simulink subsystem "rss_pmsm_motor_simscape_deltaconn"  (R2024a)
settings: Solver=VariableStepAuto  StartTime=0.0  StopTime=10.0  RelTol=1e-3
undefined symbols (not defined in the file): parMotMdlPolePairNum
libraries: nesl_utility x11, fl_lib x10, ee_lib x2, mcbcontrolslib x1
settings Model: Creator=CAV2OFO  LastModifiedBy=pav2ofo
settings OptimizationCC: ReuseModelBlockBuffer=off
settings RTWCC: GPUComputeCapability=3.5

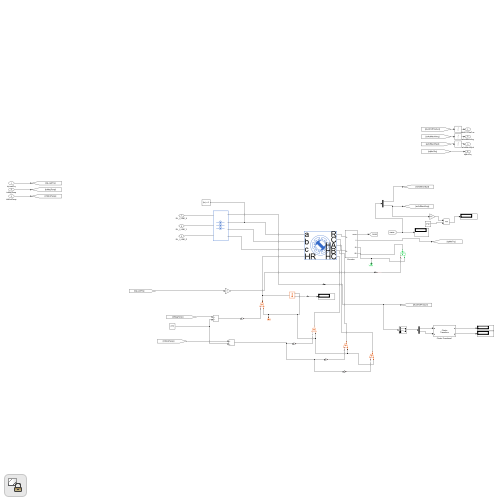
[thumbnail: Simulink's stored preview of the top-level diagram]
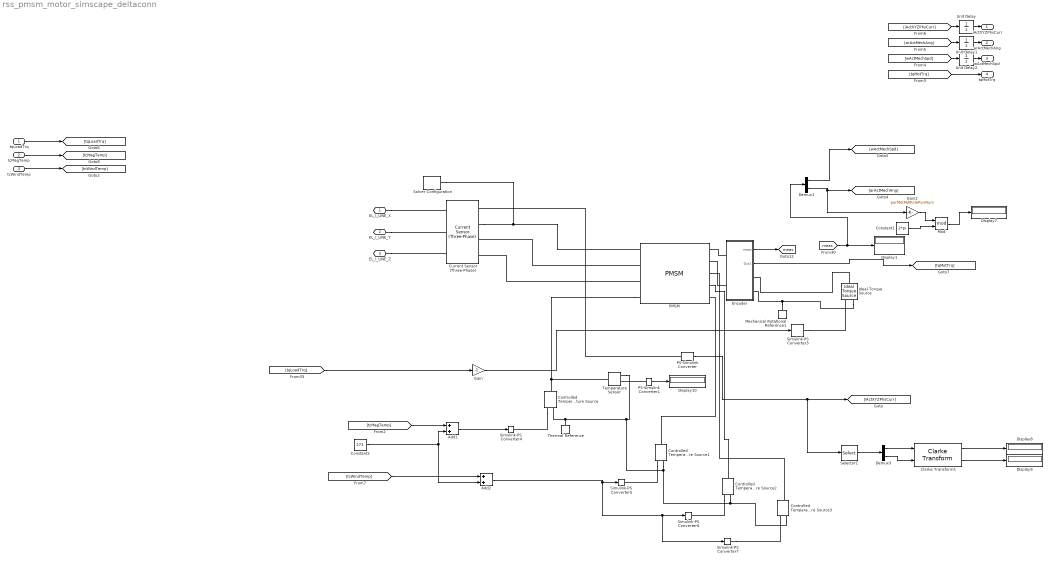
== system rss_pmsm_motor_simscape_deltaconn ==
  tqLoadTrq : Inport
  tcMagTemp : Inport  Port=2
  tcWindTemp : Inport  Port=3
  Add1 : Sum
  Add2 : Sum
  Clarke Transform1 : mcbcontrolslib/Clarke Transform  VariantControl=Variant2  PhaseInput=Two inputs  EnPowerInv=off
      settings: LibrarySourceBlock=mcbhdllib/Controls/Math Transforms/Clarke Transform
  Constant1 : Constant  Value=2*pi
  Constant2 : Constant  Value=273
  Controlled Temperature Source{,1..3} (4 alike) : fl_lib/Thermal/Thermal Sources/Controlled Temperature Source
  Current Sensor (Three-Phase) : ee_lib/Sensors & Transducers/Current Sensor (Three-Phase)
      settings: InternalSimscapePortConfiguration="{\"Bottom\":[],\"Left\":[{\"id\":\"a1\",\"label\":\"a1\",\"type\":\"foundation.electrical.electrical\"},{\"id\":\"b1\",\"label\":\"b1\",\"type\":\"foundation.electrical.electrical\"},{\"id\":\"c1\",\"label\":\"c1\",\"type\":\"foundation.electrical.electrical\"}],\"Right\":[{\"id\":\"I_output\",\"label\":\"I\",\"type\":\"output\"},{\"id\":\"a2\",\"label\":\"a2\",\"type\":\"foundation.electrical.electrical\"},{\"id\":\"b2\",\"label\":\"b2\",\"type\":\"foundation.electrical.electrical\"},{\"id\":\"c2\",\"label\":\"c2\",\"type\":\"foundation.electrical.electrical\"}],\"Top\":[]}"
  Demux1 : Demux  Outputs=2
  Demux3 : Demux  Outputs=2
  Display{1,7..10} (5 alike) : Display
  Encoder : Subsystem
  Gain : Gain  Gain=-1
  Gain2 : Gain  Gain=parMotMdlPolePairNum
  Ideal Torque Source : fl_lib/Mechanical/Mechanical Sources/Ideal Torque Source
  Mechanical Rotational Reference1 : fl_lib/Mechanical/Rotational Elements/Mechanical Rotational Reference
  Mod : Math  Operator=mod
  PMSM : ee_lib/Electromechanical/Permanent Magnet/PMSM  port_option=ee.enum.threePhasePort.expanded  winding_type=ee.enum.statorconnection.delta  machine_param=ee.enum.pmsm.parameterization.constant  nPolePairs=parMotMdlPolePairNum  pmflux_param=ee.enum.pmflux.fluxlinkage  pm_flux_linkage=parMotMdlPermMagFlux Wb  torque_constant=0.18 N*m/A  back_emf_constant=0.18 V*s/rad  stator_param=ee.enum.statorparam.LdLqL0  Ld=parMotMdlDirIndc H  Lq=parMotMdlQdrtIndc H  idVec=[-200, 0, 200] A  iqVec=[-200, 0, 200] A  LdMatrix=0.0002 * ones(3, 3) H  LqMatrix=0.0002 * ones(3, 3) H  PmMatrix=0.1 * ones(3, 3) Wb  ktMatrix=0.18 * ones(3, 3) N*m/A  keMatrix=0.18 * ones(3, 3) V*s/rad  L0=0 H  Ls=0.0002 H  Lm=-0.00002 H  Ms=0.00002 H  Rs=parMotMdlPhsRstn Ohm  zero_sequence=ee.enum.park.zerosequence.exclude  axes_param=ee.enum.rotorangle.daxis  loss_param=ee.enum.ironloss.none  losses_oc=[0, 0, 0] W  losses_sc=[0, 0, 0] W  f_losses=60 Hz  Isc_losses=95 A  J=1.652E-5 kg*m^2  lam=double(7.9577471545947675E-5)*pi/30 N*m*s/rad  i_d_specify=on  i_d_priority=None  i_d=0.1 A  i_d_nominal_specify=off  i_d_nominal_value=1  i_d_nominal_unit=A  i_q_specify=on  i_q_priority=None  i_q=0.1 A  i_q_nominal_specify=off  i_q_nominal_value=1  i_q_nominal_unit=A  torque_specify=off  torque_priority=None  torque=0 N*m  torque_nominal_specify=off  torque_nominal_value=1  torque_nominal_unit=N*m  angular_velocity_specify=off  angular_velocity_priority=High  angular_velocity=0 rpm  angular_velocity_nominal_specify=off  angular_velocity_nominal_value=1  angular_velocity_nominal_unit=rpm  angular_position_specify=off  angular_position_priority=High  angular_position=0 deg  angular_position_nominal_specify=off  angular_position_nominal_value=1  angular_position_nominal_unit=deg  alpha=parMotRstnTempCoef 1/K  alpha_flux=parMotMdlMagTempCoef 1/K  Tmeas=25 degC  stator_thermal_mass=100 J/K  rotor_thermal_mass=200 J/K  Rm_percent_rotor=90  Rd_percent_rotor=30  temperatureA_specify=on  temperatureA_priority=Low  temperatureA=25 degC  temperatureA_nominal_specify=off  temperatureA_nominal_value=1  temperatureA_nominal_unit=degC  temperatureB_specify=on  temperatureB_priority=Low  temperatureB=25 degC  temperatureB_nominal_specify=off  temperatureB_nominal_value=1  temperatureB_nominal_unit=degC  temperatureC_specify=on  temperatureC_priority=Low  temperatureC=25 degC  temperatureC_nominal_specify=off  temperatureC_nominal_value=1  temperatureC_nominal_unit=degC  temperatureR_specify=on  temperatureR_priority=Low  temperatureR=25 degC  temperatureR_nominal_specify=off  temperatureR_nominal_value=1  temperatureR_nominal_unit=degC
      settings: InternalSimscapePortConfiguration="{\"Bottom\":[],\"Left\":[{\"id\":\"a\",\"label\":\"a\",\"type\":\"foundation.electrical.electrical\"},{\"id\":\"b\",\"label\":\"b\",\"type\":\"foundation.electrical.electrical\"},{\"id\":\"c\",\"label\":\"c\",\"type\":\"foundation.electrical.electrical\"},{\"id\":\"HR\",\"label\":\"HR\",\"type\":\"foundation.thermal.thermal\"}],\"Right\":[{\"id\":\"R\",\"label\":\"R\",\"type\":\"foundation.mechanical.rotational.rotational\"},{\"id\":\"C\",\"label\":\"C\",\"type\":\"foundation.mechanical.rotational.rotational\"},{\"id\":\"HA\",\"label\":\"HA\",\"type\":\"foundation.thermal.thermal\"},{\"id\":\"HB\",\"label\":\"HB\",\"type\":\"foundation.thermal.thermal\"},{\"id\":\"HC\",\"label\":\"HC\",\"type\":\"foundation.thermal.thermal\"}],\"Top\":[]}"
  PS-Simulink Converter : nesl_utility/PS-Simulink Converter  PhysicalDomain=network_engine_domain  SubClassName=ps_output  LeftPortType=input  RightPortType=output  PseudoPeriodic=off  Frequencies=[]  VectorFormat=1-D array  Unit=A  AffineConversion=off
  PS-Simulink Converter1 : nesl_utility/PS-Simulink Converter  PhysicalDomain=network_engine_domain  SubClassName=ps_output  LeftPortType=input  RightPortType=output  PseudoPeriodic=off  Frequencies=[]  VectorFormat=inherit  Unit=inherit  AffineConversion=off
  Selector1 : Selector  InputPortWidth=3  IndexOptions=Index vector (dialog)  Indices=[1 2]  OutputSizes=1
  Simulink-PS Converter3 : nesl_utility/Simulink-PS Converter  PhysicalDomain=network_engine_domain  SubClassName=ps_input  LeftPortType=input  RightPortType=output  PseudoPeriodic=off  Frequencies=[]  NoiseDistribution=none  NoiseParameters=[]  Unit=1  AffineConversion=off  FilteringAndDerivatives=zero  SimscapeFilterOrder=1  InputFilterTimeConstant=.001  UdotUserProvided=0
  Simulink-PS Converter{4..7} (4 alike) : nesl_utility/Simulink-PS Converter  PhysicalDomain=network_engine_domain  SubClassName=ps_input  LeftPortType=input  RightPortType=output  PseudoPeriodic=off  Frequencies=[]  NoiseDistribution=none  NoiseParameters=[]  Unit=1  AffineConversion=off  FilteringAndDerivatives=filter  SimscapeFilterOrder=1  InputFilterTimeConstant=0.001  UdotUserProvided=0
  Solver Configuration : nesl_utility/Solver Configuration  PhysicalDomain=network_engine_domain  SubClassName=solver  LeftPortType=input  RightPortType=generic  Tones=[]  Harmonics=[]  SimulateNoise=off  Profile=off  UseLocalSampling=off  EnableSwitchedLinearOptims=on  FrequencyDomain=off  UseCCode=off  RelTol=0.001  AbsTol=0.001  MinStep=1e-09  ToWorkspace=off  RevertToSquareIcSolve=off  NumHomotopyIterations=100  PhasorMode=off  PhasorModeNumHarmonics=1  ConsistencySolver=NEWTON_XTOL_AFTER_FTOL  IndexReductionMethod=DerivativeReplacement  DoDC=off  ResidualTolerance=1e-09  ConsistencyTolSource=GLOBAL  ConsistencyAbsTol=0.001  ConsistencyRelTol=0.001  ConsistencyTolFactor=0.001  UseLocalSolver=on  LocalSolverChoice=NE_BACKWARD_EULER_ADVANCER  ResolveIndetEquations=on  FunctionEvalNumThread=1  LocalSolverSampleTime=cstMotorMdlSampTime  DoFixedCost=on  MaxNonlinIter=3  MaxModeIter=2  ComputeImpulses=off  ImpulseIterations=2  LinearAlgebra=auto  LinearAlgebraNumThread=0  EquationFormulation=NE_TIME_EF  DelaysMemoryBudget=1024  AutomaticFiltering=on  FilteringTimeConstant=0.001  PartitionStorageMethod=AS_NEEDED  PartitionMemoryBudget=1024  PartitionMethod=ROBUST  MultibodyUseLocalSolver=off  MultibodyLocalSolverChoice=ODE1  MultibodyLocalSolverSampleTime=0.001
  Temperature Sensor : fl_lib/Thermal/Thermal Sensors/Temperature Sensor  temperature_measure=foundation.enum.MeasurementReference.difference
  Thermal Reference : fl_lib/Thermal/Thermal Elements/Thermal Reference
  Unit Delay : UnitDelay  SampleTime=-1  HasFrameUpgradeWarning=on
  Unit Delay1 : UnitDelay  SampleTime=-1  HasFrameUpgradeWarning=on
  Unit Delay2 : UnitDelay  SampleTime=-1  HasFrameUpgradeWarning=on
  EL_I_LINE_X : PMIOPort  Side=Left
  EL_I_LINE_Y : PMIOPort  Port=2  Side=Left
  EL_I_LINE_Z : PMIOPort  Port=3  Side=Left
  iActXYZPhsCurr : Outport
  arActMechAng : Outport  Port=2
  wActMechSpd : Outport  Port=3
  tqMotTrq : Outport  Port=4
  tag scope: meas=global
  wires:
  Encoder/1(meas) -> [meas]
  Add2/1 -> Simulink-PS Converter7/1, Simulink-PS Converter6/1, Simulink-PS Converter5/1
  Clarke Transform1/1 -> Display8/1
  [tqMotTrq] -> tqMotTrq/1
  tqLoadTrq/1 -> [tqLoadTrq]
  Mod/1 -> Display7/1
  Constant2/1 -> Add2/2, Add1/2
  tcMagTemp/1 -> [tcMagTemp]
  [tcWindTemp] -> Add2/1
  Clarke Transform1/2 -> Display9/1
  Unit Delay1/1 -> arActMechAng/1
  Add1/1 -> Simulink-PS Converter4/1
  Gain/1 -> Simulink-PS Converter3/1
  Demux1/1 -> [wActMechSpd]
  PS-Simulink Converter1/1 -> Display10/1
  Unit Delay2/1 -> wActMechSpd/1
  Encoder/2(Out1) -> [tqMotTrq]
  tcWindTemp/1 -> [tcWindTemp]
  Demux1/2 -> Gain2/1, [arActMechAng]
  Unit Delay/1 -> iActXYZPhsCurr/1
  Constant1/1 -> Mod/2
  Gain2/1 -> Mod/1
  [tcMagTemp] -> Add1/1
  Demux3/1 -> Clarke Transform1/1
  Demux3/2 -> Clarke Transform1/2
  PS-Simulink Converter/1 -> Selector1/1, [iActXYZPhsCurr]
  [meas] -> Demux1/1, Display1/1
  [arActMechAng] -> Unit Delay1/1
  [tqLoadTrq] -> Gain/1
  [iActXYZPhsCurr] -> Unit Delay/1
  Selector1/1 -> Demux3/1
  [wActMechSpd] -> Unit Delay2/1
  connections:
  Controlled Temperature Source3/RConn2 -- Thermal Reference/LConn1 -- Controlled Temperature Source/RConn2 -- Temperature Sensor/RConn1 -- Controlled Temperature Source1/RConn2 -- Controlled Temperature Source2/RConn2
  PMSM/LConn4 -- Temperature Sensor/LConn1 -- Controlled Temperature Source/LConn1
  Mechanical Rotational Reference1/LConn1 -- Encoder/RConn2 -- Ideal Torque Source/RConn2
  Solver Configuration/RConn1 -- Current Sensor (Three-Phase)/RConn2 -- PMSM/LConn1
  Controlled Temperature Source/RConn1 -- Simulink-PS Converter4/RConn1
  PMSM/LConn2 -- Current Sensor (Three-Phase)/RConn3
  PMSM/RConn4 -- Controlled Temperature Source2/LConn1
  Controlled Temperature Source1/LConn1 -- PMSM/RConn5
  Simulink-PS Converter7/RConn1 -- Controlled Temperature Source3/RConn1
  Controlled Temperature Source3/LConn1 -- PMSM/RConn3
  Controlled Temperature Source2/RConn1 -- Simulink-PS Converter6/RConn1
  PS-Simulink Converter/LConn1 -- Current Sensor (Three-Phase)/RConn1
  Controlled Temperature Source1/RConn1 -- Simulink-PS Converter5/RConn1
  Ideal Torque Source/LConn1 -- Encoder/RConn1
  Simulink-PS Converter3/RConn1 -- Ideal Torque Source/RConn1
  PMSM/LConn3 -- Current Sensor (Three-Phase)/RConn4
  Encoder/LConn2 -- PMSM/RConn2
  Encoder/LConn1 -- PMSM/RConn1
  PS-Simulink Converter1/LConn1 -- Temperature Sensor/RConn2
  EL_I_LINE_Z/RConn1 -- Current Sensor (Three-Phase)/LConn3
  EL_I_LINE_X/RConn1 -- Current Sensor (Three-Phase)/LConn1
  EL_I_LINE_Y/RConn1 -- Current Sensor (Three-Phase)/LConn2

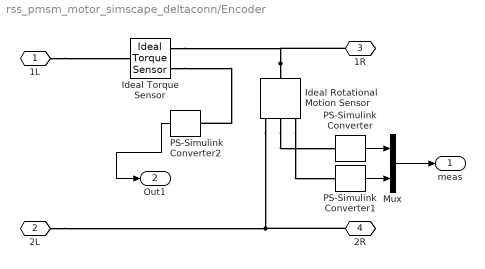
== system rss_pmsm_motor_simscape_deltaconn/Encoder ==
  Ideal Rotational Motion Sensor : fl_lib/Mechanical/Mechanical Sensors/Ideal Rotational Motion Sensor  reference=foundation.enum.MeasurementReference.difference  acceleration_port=false  velocity_port=true  position_port=true  wrap_angle=true  offset=0 deg
  Ideal Torque Sensor : fl_lib/Mechanical/Mechanical Sensors/Ideal Torque Sensor
  Mux : Mux  Inputs=2
  PS-Simulink Converter : nesl_utility/PS-Simulink Converter  PhysicalDomain=network_engine_domain  SubClassName=ps_output  LeftPortType=input  RightPortType=output  PseudoPeriodic=off  Frequencies=[]  VectorFormat=1-D array  Unit=rad/s  AffineConversion=off
  PS-Simulink Converter1 : nesl_utility/PS-Simulink Converter  PhysicalDomain=network_engine_domain  SubClassName=ps_output  LeftPortType=input  RightPortType=output  PseudoPeriodic=off  Frequencies=[]  VectorFormat=1-D array  Unit=rad  AffineConversion=off
  PS-Simulink Converter2 : nesl_utility/PS-Simulink Converter  PhysicalDomain=network_engine_domain  SubClassName=ps_output  LeftPortType=input  RightPortType=output  PseudoPeriodic=off  Frequencies=[]  VectorFormat=1-D array  Unit=N*m  AffineConversion=off
  1L : PMIOPort  Side=Left
  2L : PMIOPort  Port=2  Side=Left
  1R : PMIOPort  Port=3  Side=Right
  2R : PMIOPort  Port=4  Side=Right
  meas : Outport  VectorParamsAs1DForOutWhenUnconnected=off
  Out1 : Outport  Port=2
  wires:
  PS-Simulink Converter2/1 -> Out1/1
  Mux/1 -> meas/1
  PS-Simulink Converter1/1 -> Mux/2
  PS-Simulink Converter/1 -> Mux/1
  connections:
  Ideal Torque Sensor/RConn2 -- PS-Simulink Converter2/LConn1
  1L/RConn1 -- Ideal Torque Sensor/LConn1
  2R/RConn1 -- 2L/RConn1 -- Ideal Rotational Motion Sensor/RConn1
  Ideal Rotational Motion Sensor/LConn1 -- 1R/RConn1 -- Ideal Torque Sensor/RConn1
  Ideal Rotational Motion Sensor/RConn2 -- PS-Simulink Converter/LConn1
  Ideal Rotational Motion Sensor/RConn3 -- PS-Simulink Converter1/LConn1
